simulink model "TP09_Ej09"  (R2020b)
settings: Solver=FixedStepAuto  StartTime=0.0  StopTime=5  FixedStep=1e-3  RelTol=1e-3  EnableMultiTasking=on
settings Model: Creator=54115  LastModifiedBy=Juan
settings DataIOCC: ReturnWorkspaceOutputs=off
settings OptimizationCC: LifeSpan=inf
settings DebuggingCC: SFUnexpectedBacktrackingDiag=warning  SFNoUnconditionalDefaultTransitionDiag=warning  ArithmeticOperatorsInVariantConditions=warning
settings SFSimCC: SimUseLocalCustomCode=off  CustomCodeUndefinedFunction=UseInterfaceOnly
settings RTWCC: RTWUseLocalCustomCode=off
settings CodeAppCC: StateflowObjectComments=on
settings GRTTargetCC: TargetLangStandard=C89/C90 (ANSI)
settings ConfigComp: CovMetricSettings=dw  CovSaveCumulativeToWorkspaceVar=on  CovSaveSingleToWorkspaceVar=on  CovExternalEMLEnable=off

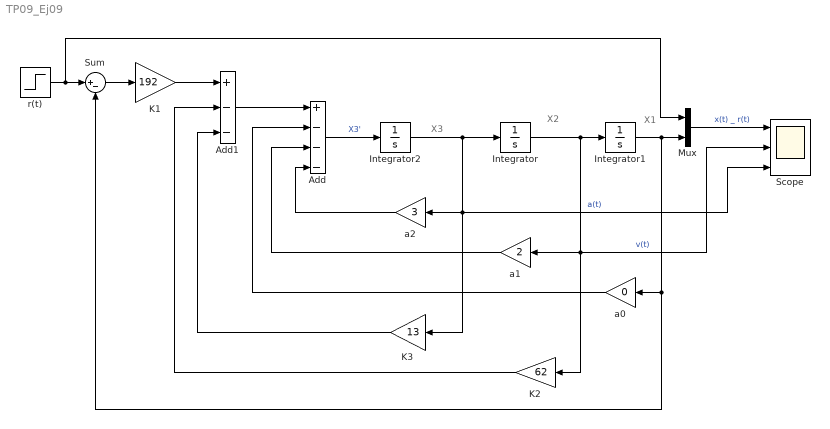
== system TP09_Ej09 ==
  note: X1
  note: X2
  note: X3
  Add : Sum  Inputs=+---
  Add1 : Sum  Inputs=+--
  Integrator : Integrator
  Integrator1 : Integrator
  Integrator2 : Integrator
  K1 : Gain  Gain=192
  K2 : Gain  Gain=62
  K3 : Gain  Gain=13
  Mux : Mux  Inputs=2
  Scope : Scope  NumInputPorts=3
  Sum : Sum  Inputs=|+-
  a0 : Gain  Gain=0
  a1 : Gain  Gain=2
  a2 : Gain  Gain=3
  r(t) : Step  Time=0  SampleTime=0
  wires:
  Integrator2/1 -> Integrator/1, K3/1, Scope/3, a2/1  "a(t)"
  Integrator/1 -> Scope/2, K2/1, a1/1, Integrator1/1  "v(t)"
  Add/1 -> Integrator2/1  "X3'"
  Integrator1/1 -> Mux/2, Sum/2, a0/1
  Mux/1 -> Scope/1  "x(t) _ r(t)"
  Add1/1 -> Add/1
  K1/1 -> Add1/1
  K3/1 -> Add1/3
  K2/1 -> Add1/2
  r(t)/1 -> Mux/1, Sum/1
  Sum/1 -> K1/1
  a2/1 -> Add/4
  a1/1 -> Add/3
  a0/1 -> Add/2
